simulink model "Q2_Karnopp"  (R2016b)
settings: Solver=VariableStepAuto  StartTime=0.0  StopTime=10.0  RelTol=1e-3
values from neighbouring files (symbols this model uses):
  c_a = 0.1    [CSD_HW_1_Script.m]
  D_v = 1e-2    (= 0.01)    [CSD_HW_1_Script.m]
  J = 0.07    [CSD_HW_1_Script.m]
  K_t = 0.46    [CSD_HW_1_Script.m]
  l = 0.3    [CSD_HW_1_Script.m]
  m = 0.8    [CSD_HW_1_Script.m]
  N = 3    [Plotshit.m]
  R = 0.76    [CSD_HW_1_Script.m]    (also in Plotshit.m = 0.1)
  V_max = 20    [CSD_HW_1_Script.m]
undefined symbols (not defined in the file or in its folder): magnitude, T_sl, T_st
libraries: cstblocks x1
settings Model: Creator=nadav  LastModifiedBy=nadav

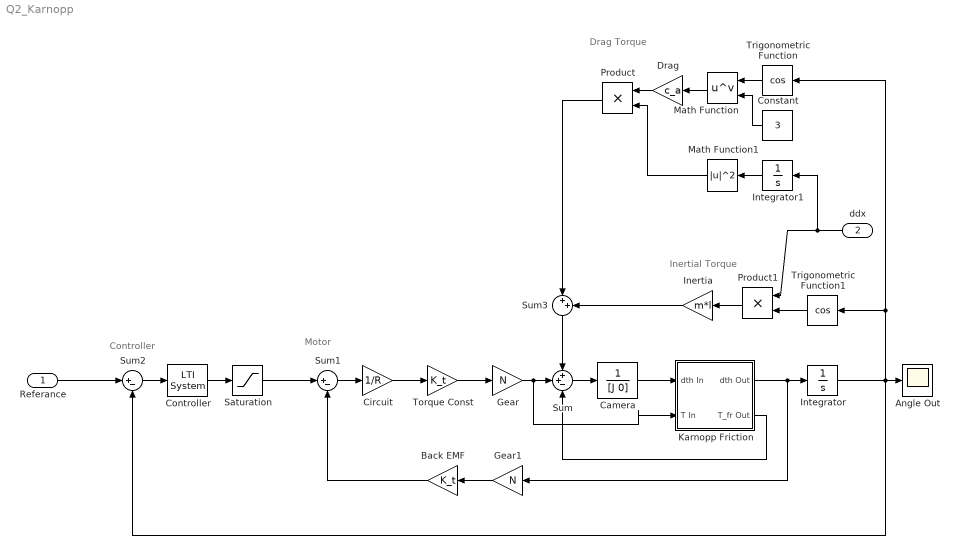
== system Q2_Karnopp ==
  note: Inertial Torque
  note: Drag Torque
  note: Controller
  note: Motor
  Referance : Inport
  ddx : Inport  Port=2
  Angle Out : Scope
  Back EMF : Gain  Gain=K_t
  Camera : TransferFcn  Denominator=[J 0]
  Circuit : Gain  Gain=1/R
  Constant : Constant  Value=3
  Controller : cstblocks/LTI System  sys=C  IC=[]
  Drag : Gain  Gain=c_a
  Gear : Gain  Gain=N
  Gear1 : Gain  Gain=N
  Inertia : Gain  Gain=m*l
  Integrator : Integrator
  Integrator1 : Integrator
  Karnopp Friction : Subsystem
  Math Function : Math  Operator=pow  SaturateOnIntegerOverflow=on
  Math Function1 : Math  Operator=magnitude^2  SaturateOnIntegerOverflow=on
  Product : Product
  Product1 : Product
  Saturation : Saturate  UpperLimit=V_max  LowerLimit=-V_max
  Sum : Sum  Inputs=++-
  Sum1 : Sum  Inputs=|+-
  Sum2 : Sum  Inputs=|+-
  Sum3 : Sum  Inputs=|++
  Torque Const : Gain  Gain=K_t
  Trigonometric Function : Trigonometry  Operator=cos
  Trigonometric Function1 : Trigonometry  Operator=cos
  wires:
  Karnopp Friction/1(dth Out) -> Gear1/1, Integrator/1
  Camera/1 -> Karnopp Friction/1(dth In)
  Sum/1 -> Camera/1
  Gear/1 -> Sum/2, Karnopp Friction/2(T In)
  Karnopp Friction/2(T_fr Out) -> Sum/3
  Torque Const/1 -> Gear/1
  Circuit/1 -> Torque Const/1
  Gear1/1 -> Back EMF/1
  Back EMF/1 -> Sum1/2
  Sum1/1 -> Circuit/1
  Sum2/1 -> Controller/1
  Integrator/1 -> Sum2/2, Trigonometric Function1/1, Trigonometric Function/1, Angle Out/1
  Saturation/1 -> Sum1/1
  Controller/1 -> Saturation/1
  Referance/1 -> Sum2/1
  ddx/1 -> Product1/1, Integrator1/1
  Trigonometric Function/1 -> Math Function/1
  Constant/1 -> Math Function/2
  Math Function/1 -> Drag/1
  Integrator1/1 -> Math Function1/1
  Sum3/1 -> Sum/1
  Drag/1 -> Product/1
  Math Function1/1 -> Product/2
  Product/1 -> Sum3/1
  Trigonometric Function1/1 -> Product1/2
  Product1/1 -> Inertia/1
  Inertia/1 -> Sum3/2

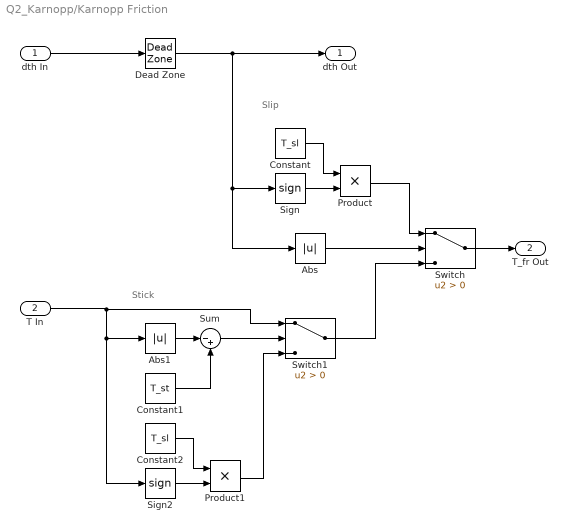
== system Q2_Karnopp/Karnopp Friction ==
  note: Stick
  note: Slip
  dth In : Inport
  T In : Inport  Port=2
  Abs : Abs
  Abs1 : Abs
  Constant : Constant  Value=T_sl
  Constant1 : Constant  Value=T_st
  Constant2 : Constant  Value=T_sl
  Dead Zone : DeadZone  LowerValue=-D_v/2  UpperValue=D_v/2  SaturateOnIntegerOverflow=on
  Product : Product
  Product1 : Product
  Sign : Signum
  Sign2 : Signum
  Sum : Sum  Inputs=|-+
  Switch : Switch  Criteria=u2 > Threshold
  Switch1 : Switch  Criteria=u2 > Threshold
  dth Out : Outport
  T_fr Out : Outport  Port=2
  wires:
  Product/1 -> Switch/1
  Sum/1 -> Switch1/2
  Constant1/1 -> Sum/2
  Abs1/1 -> Sum/1
  Constant/1 -> Product/1
  Sign/1 -> Product/2
  T In/1 -> Sign2/1, Abs1/1, Switch1/1
  Sign2/1 -> Product1/2
  Product1/1 -> Switch1/3
  Abs/1 -> Switch/2
  dth In/1 -> Dead Zone/1
  Constant2/1 -> Product1/1
  Switch1/1 -> Switch/3
  Dead Zone/1 -> dth Out/1, Abs/1, Sign/1
  Switch/1 -> T_fr Out/1
